simulink model "Satellite_formation_control"  (R2020b)
settings: Solver=VariableStepAuto  StartTime=0.0  StopTime=run_time  RelTol=1e-3
values from neighbouring files (symbols this model uses):
  A = [zeros(3) eye(3) ... (first row only)    [Dynamic_output_feedback_formation_control.m]    (also in Robust_consensus.m; Robust_consensus_S_procedure.m; Robust_consensus_against_model_uncertainty.m; Stable_Consensus.m)
  Am = kron(eye(N),A)    [Robust_consensus.m]    (also in Robust_consensus_S_procedure.m = blkdiag(A,(1+delta2)*A, (1+delta3)*A, (1+delta4)*A, (1+delta; Robust_consensus_against_model_uncertainty.m = blkdiag(A,A+Delta2, A+Delta3, A+Delta4, A+Delta5, A+Delta6); Stable_Consensus.m; alpha_stability.m = blkdiag(A,A+Delta2, A+Delta3, A+Delta4, A+Delta5, A+Delta6))
  Amp = 1    [Frequency_experiment.m]
  Bm = kron(eye(N),B)    [Robust_consensus.m]    (also in Robust_consensus_S_procedure.m; Robust_consensus_against_model_uncertainty.m; Stable_Consensus.m; alpha_stability.m)
  Cm = kron(eye(N),C)    [output_feedback_formation_control.m]
  D = kron(I_tilde,ones(n,1))    [Robust_consensus.m]    (also in Robust_consensus_S_procedure.m; Robust_consensus_against_model_uncertainty.m; Stable_Consensus.m; alpha_stability.m)
  delta2 = 0.5    [Robust_consensus.m]    (also in Robust_consensus_S_procedure.m)
  delta3 = 0.1    [Robust_consensus.m]    (also in Robust_consensus_S_procedure.m)
  delta4 = 0.07    [Robust_consensus.m]    (also in Robust_consensus_S_procedure.m)
  delta5 = 0.03    [Robust_consensus.m]    (also in Robust_consensus_S_procedure.m)
  delta6 = 0.09    [Robust_consensus.m]    (also in Robust_consensus_S_procedure.m)
  freq = Freq(iter)    [Frequency_experiment.m]
  gamma = 2.1    [Dynamic_output_feedback_formation_control.m]    (also in Robust_consensus.m = sqrt(4/alpha); Robust_consensus_S_procedure.m = sqrt(alpha); Robust_consensus_against_model_uncertainty.m = 2*sqrt(alpha); alpha_stability.m = 0.1)
  Km = kron(L,-c*B*K)    [Robust_consensus.m]    (also in Robust_consensus_S_procedure.m; Robust_consensus_against_model_uncertainty.m; Stable_Consensus.m; alpha_stability.m = kron(L,c*B*K))
  Um = kron(U,eye(n))    [Robust_consensus.m]    (also in Robust_consensus_S_procedure.m = kron(inv(U),eye(n)); alpha_stability.m = kron(inv(U),eye(n)))
  x0 = [x1_0 ... (first row only)    [Robust_consensus.m]    (also in Robust_consensus_S_procedure.m; Robust_consensus_against_model_uncertainty.m; Stable_Consensus.m; alpha_stability.m)
  x1_0 = [0 500 866*sqrt(3) 1.5 0 0].'    [Robust_consensus.m]    (also in Robust_consensus_S_procedure.m; Robust_consensus_against_model_uncertainty.m; Stable_Consensus.m; alpha_stability.m)
  x1dm = kron(ones(N,1),x1d)    [Robust_consensus.m]    (also in Robust_consensus_S_procedure.m; Robust_consensus_against_model_uncertainty.m; alpha_stability.m)
  xd = [x1d ... (first row only)    [Robust_consensus.m]    (also in Robust_consensus_S_procedure.m; Robust_consensus_against_model_uncertainty.m; Stable_Consensus.m; alpha_stability.m)
settings Model: Creator=yu zheng  LastModifiedBy=yu zheng

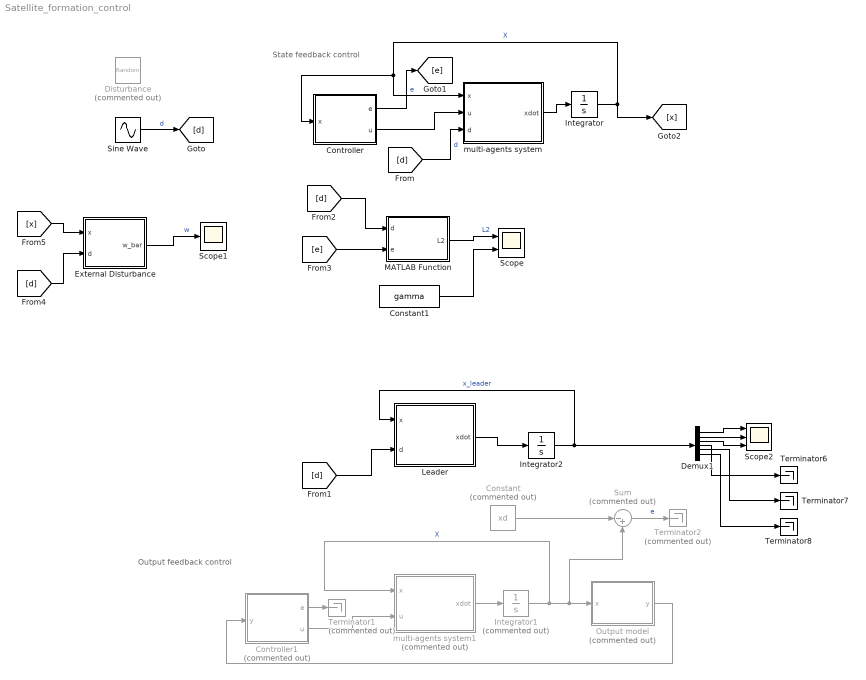
== system Satellite_formation_control ==
  note: State feedback control
  note: Output feedback control
  Constant : Constant  Commented=on  Value=xd
  Constant1 : Constant  Value=gamma
  Controller : MATLAB Function  TreatAsAtomicUnit=on
  Controller1 : MATLAB Function  Commented=on  TreatAsAtomicUnit=on
  Demux1 : Demux  Outputs=6
  Disturbance : RandomNumber  Commented=on  Variance=4  SampleTime=0.1
  External Disturbance : MATLAB Function  TreatAsAtomicUnit=on
  Integrator : Integrator  InitialCondition=x0
  Integrator1 : Integrator  Commented=on  InitialCondition=x0
  Integrator2 : Integrator  InitialCondition=x1_0
  Leader : MATLAB Function  TreatAsAtomicUnit=on
  MATLAB Function : MATLAB Function  TreatAsAtomicUnit=on
  Output model : MATLAB Function  Commented=on  TreatAsAtomicUnit=on
  Scope : Scope  NumInputPorts=2
  Scope1 : Scope
  Scope2 : Scope  NumInputPorts=3
  Sine Wave : Sin  Amplitude=Amp  Frequency=freq  SampleTime=0
  Sum : Sum  Commented=on  Inputs=|-+
  Terminator1 : Terminator  Commented=on
  Terminator2 : Terminator  Commented=on
  Terminator6 : Terminator
  Terminator7 : Terminator
  Terminator8 : Terminator
  multi-agents system : MATLAB Function  TreatAsAtomicUnit=on
  multi-agents system1 : MATLAB Function  Commented=on  TreatAsAtomicUnit=on
  wires:
  multi-agents system/1(xdot) -> Integrator/1
  Integrator/1 -> [x], Controller/1(x), multi-agents system/1(x)  "X"
  Controller/2(u) -> multi-agents system/2(u)
  Controller/1(e) -> [e]  "e"
  multi-agents system1/1(xdot) -> Integrator1/1
  Controller1/2(u) -> multi-agents system1/2(u)
  Integrator1/1 -> Sum/2, Output model/1(x), multi-agents system1/1(x)  "X"
  Controller1/1(e) -> Terminator1/1
  Output model/1(y) -> Controller1/1(y)
  Constant/1 -> Sum/1
  Sum/1 -> Terminator2/1  "e"
  Leader/1(xdot) -> Integrator2/1
  [d] -> Leader/2(d)
  Demux1/4 -> Terminator6/1
  Demux1/1 -> Scope2/1
  Demux1/2 -> Scope2/2
  Integrator2/1 -> Leader/1(x), Demux1/1  "x_leader"
  Demux1/3 -> Scope2/3
  Demux1/6 -> Terminator8/1
  Demux1/5 -> Terminator7/1
  [d] -> multi-agents system/3(d)  "d"
  Sine Wave/1 -> [d]  "d"
  [d] -> MATLAB Function/1(d)
  [e] -> MATLAB Function/2(e)
  MATLAB Function/1(L2) -> Scope/1  "L2"
  Constant1/1 -> Scope/2
  [x] -> External Disturbance/1(x)
  [d] -> External Disturbance/2(d)
  External Disturbance/1(w_bar) -> Scope1/1  "w"

== matlab function Satellite_formation_control/Controller ==
  data: e output; x input; u output; xd parameter; Km parameter; Am parameter; x1dm parameter
function [e,u] = fcn(x,xd,Km,Am,x1dm)

% x1 = x(1:n);
% x2 = x(n+1:2*n);
% x3 = x(2*n+1:3*n);
% x4 = x(3*n+1:4*n);
% x5 = x(4*n+1:5*n);
% x6 = x(5*n+1:6*n);

% e = Um*(x-xd);
e = x-xd;
u = -Am*(xd-x1dm) + Km*(x-xd);
u(1:6)=zeros(6,1);

== matlab function Satellite_formation_control/multi-agents system ==
  data: x input; u input; xdot output; Am parameter; d input; D parameter
function xdot = fcn(x,u,Am, d,D)


xdot = Am*x +u + D*d;

== matlab function Satellite_formation_control/Controller1 ==
  data: e output; y input; u output; xd parameter; Km parameter; Am parameter; Cm parameter
function [e,u] = fcn(y,xd,Km,Am,Cm)

% x1 = x(1:n);
% x2 = x(n+1:2*n);
% x3 = x(2*n+1:3*n);
% x4 = x(3*n+1:4*n);
% x5 = x(4*n+1:5*n);
% x6 = x(5*n+1:6*n);

e = y-Cm*xd;
u = -Am*xd + Km*e;
u(1:6)=zeros(6,1);

== matlab function Satellite_formation_control/multi-agents system1 ==
  data: x input; u input; xdot output; Am parameter; Bm parameter
function xdot = fcn(x,u,Am, Bm)

xdot = Am*x +u;

== matlab function Satellite_formation_control/Output model ==
  data: x input; y output; Cm parameter
function y = fcn(x,Cm)

y = Cm*x;

== matlab function Satellite_formation_control/MATLAB Function ==
  data: d input; L2 output; e input; gamma parameter
function L2 = fcn(d,e, gamma)


e12 = norm(-e(1:6)+e(7:12));
L2 = e12/norm(d);

== matlab function Satellite_formation_control/Leader ==
  data: x input; xdot output; d input; A parameter
function xdot = fcn(x,d, A)

n = size(A,1);
xdot = A*x  + ones(n,1)*d;

== matlab function Satellite_formation_control/External Disturbance ==
  data: x input; w_bar output; d input; delta2 parameter; delta3 parameter; delta4 parameter; delta5 parameter; delta6 parameter; Um parameter; A parameter
function w_bar = fcn(x,d,delta2, delta3, delta4, delta5, delta6,Um, A)

x1 = x(1:6);
w1 = d*ones(6,1);

w2 = delta2*A*x1-w1;
w3 = delta3*A*x1-w1;
w4 = delta4*A*x1-w1;
w5 = delta5*A*x1-w1;
w6 = delta6*A*x1-w1;

w = [zeros(6,1); w2; w3; w4; w5; w6];
w_bar = Um*w;
